simulink model "hw2Q6_model"  (R2021a)
settings: Solver=VariableStepAuto  StartTime=0.0  StopTime=time_end  RelTol=1e-3
settings Model: Creator=kaiyu  LastModifiedBy=kaiyu

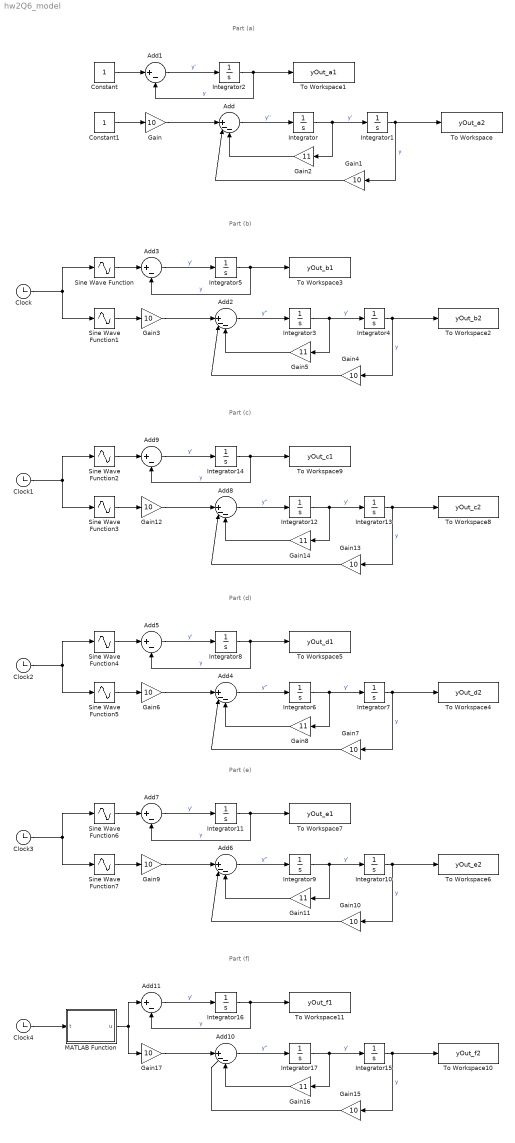
== system hw2Q6_model ==
  note: Part (a)
  note: Part (b)
  note: Part (d)
  note: Part (e)
  note: Part (c)
  note: Part (f)
  Add{,2,4,6,8,10} (6 alike) : Sum  Inputs=||+--
  Add{1,3,5,7,9,11} (6 alike) : Sum  Inputs=|+-
  Clock{,1..4} (5 alike) : Clock
  Constant : Constant
  Constant1 : Constant
  Gain{,1,3..4,6..7,9..10,12..13,15,17} (12 alike) : Gain  Gain=10
  Gain{2,5,8,11,14,16} (6 alike) : Gain  Gain=11
  Integrator{,1..17} (18 alike) : Integrator
  MATLAB Function : MATLAB Function  TreatAsAtomicUnit=on
  Sine Wave Function : Sin  TimeSource=Use external signal  SampleTime=0
  Sine Wave Function1 : Sin  TimeSource=Use external signal  SampleTime=0
  Sine Wave Function2 : Sin  TimeSource=Use external signal  Frequency=5  Phase=pi / 2  SampleTime=0
  Sine Wave Function3 : Sin  TimeSource=Use external signal  Frequency=5  Phase=pi / 2  SampleTime=0
  Sine Wave Function4 : Sin  TimeSource=Use external signal  Amplitude=25  Frequency=10  Phase=pi / 2  SampleTime=0
  Sine Wave Function5 : Sin  TimeSource=Use external signal  Amplitude=25  Frequency=10  Phase=pi / 2  SampleTime=0
  Sine Wave Function6 : Sin  TimeSource=Use external signal  Amplitude=25  Frequency=20  Phase=pi / 2  SampleTime=0
  Sine Wave Function7 : Sin  TimeSource=Use external signal  Amplitude=25  Frequency=20  Phase=pi / 2  SampleTime=0
  To Workspace : ToWorkspace  VariableName=yOut_a2  SaveFormat=Timeseries  SampleTime=-1
  To Workspace1 : ToWorkspace  VariableName=yOut_a1  SaveFormat=Timeseries  SampleTime=-1
  To Workspace10 : ToWorkspace  VariableName=yOut_f2  SaveFormat=Timeseries  SampleTime=-1
  To Workspace11 : ToWorkspace  VariableName=yOut_f1  SaveFormat=Timeseries  SampleTime=-1
  To Workspace2 : ToWorkspace  VariableName=yOut_b2  SaveFormat=Timeseries  SampleTime=-1
  To Workspace3 : ToWorkspace  VariableName=yOut_b1  SaveFormat=Timeseries  SampleTime=-1
  To Workspace4 : ToWorkspace  VariableName=yOut_d2  SaveFormat=Timeseries  SampleTime=-1
  To Workspace5 : ToWorkspace  VariableName=yOut_d1  SaveFormat=Timeseries  SampleTime=-1
  To Workspace6 : ToWorkspace  VariableName=yOut_e2  SaveFormat=Timeseries  SampleTime=-1
  To Workspace7 : ToWorkspace  VariableName=yOut_e1  SaveFormat=Timeseries  SampleTime=-1
  To Workspace8 : ToWorkspace  VariableName=yOut_c2  SaveFormat=Timeseries  SampleTime=-1
  To Workspace9 : ToWorkspace  VariableName=yOut_c1  SaveFormat=Timeseries  SampleTime=-1
  wires:
  Gain/1 -> Add/1
  Add/1 -> Integrator/1  "y''"
  Integrator/1 -> Gain2/1, Integrator1/1  "y'"
  Integrator1/1 -> Gain1/1, To Workspace/1  "y"
  Gain1/1 -> Add/2
  Gain2/1 -> Add/3
  Add1/1 -> Integrator2/1  "y'"
  Integrator2/1 -> Add1/2, To Workspace1/1  "y"
  Add3/1 -> Integrator5/1  "y'"
  Gain5/1 -> Add2/3
  Integrator4/1 -> Gain4/1, To Workspace2/1  "y"
  Integrator5/1 -> Add3/2, To Workspace3/1  "y"
  Gain4/1 -> Add2/2
  Gain3/1 -> Add2/1
  Integrator3/1 -> Gain5/1, Integrator4/1  "y'"
  Add2/1 -> Integrator3/1  "y''"
  Constant/1 -> Add1/1
  Constant1/1 -> Gain/1
  Gain7/1 -> Add4/2
  Integrator6/1 -> Gain8/1, Integrator7/1  "y'"
  Gain6/1 -> Add4/1
  Integrator8/1 -> Add5/2, To Workspace5/1  "y"
  Add4/1 -> Integrator6/1  "y''"
  Integrator7/1 -> Gain7/1, To Workspace4/1  "y"
  Gain8/1 -> Add4/3
  Add5/1 -> Integrator8/1  "y'"
  Add6/1 -> Integrator9/1  "y''"
  Integrator11/1 -> Add7/2, To Workspace7/1  "y"
  Gain9/1 -> Add6/1
  Add7/1 -> Integrator11/1  "y'"
  Gain10/1 -> Add6/2
  Integrator10/1 -> Gain10/1, To Workspace6/1  "y"
  Integrator9/1 -> Gain11/1, Integrator10/1  "y'"
  Gain11/1 -> Add6/3
  Add8/1 -> Integrator12/1  "y''"
  Integrator14/1 -> Add9/2, To Workspace9/1  "y"
  Gain12/1 -> Add8/1
  Add9/1 -> Integrator14/1  "y'"
  Gain13/1 -> Add8/2
  Integrator13/1 -> Gain13/1, To Workspace8/1  "y"
  Integrator12/1 -> Gain14/1, Integrator13/1  "y'"
  Gain14/1 -> Add8/3
  Integrator17/1 -> Gain16/1, Integrator15/1  "y'"
  Gain16/1 -> Add10/3
  Integrator15/1 -> Gain15/1, To Workspace10/1  "y"
  Gain17/1 -> Add10/1
  Add11/1 -> Integrator16/1  "y'"
  Integrator16/1 -> Add11/2, To Workspace11/1  "y"
  Gain15/1 -> Add10/2
  Add10/1 -> Integrator17/1  "y''"
  Sine Wave Function/1 -> Add3/1
  Sine Wave Function1/1 -> Gain3/1
  Clock/1 -> Sine Wave Function/1, Sine Wave Function1/1
  Sine Wave Function2/1 -> Add9/1
  Sine Wave Function3/1 -> Gain12/1
  Clock1/1 -> Sine Wave Function2/1, Sine Wave Function3/1
  Sine Wave Function4/1 -> Add5/1
  Sine Wave Function5/1 -> Gain6/1
  Clock2/1 -> Sine Wave Function5/1, Sine Wave Function4/1
  Sine Wave Function6/1 -> Add7/1
  Sine Wave Function7/1 -> Gain9/1
  Clock3/1 -> Sine Wave Function7/1, Sine Wave Function6/1
  MATLAB Function/1(u) -> Add11/1, Gain17/1
  Clock4/1 -> MATLAB Function/1(t)

== matlab function hw2Q6_model/MATLAB Function ==
  data: t input; u output
function u = hw2Q6_f_func(t)
if (0 <= t) && (t < 3)
    input = t;

elseif (3 <= t) && (t < 5)
    input = 3;

elseif (5 <= t) && (t < 7)
    input = -3;
    
else
    input = 2 * t - 17;
end

u = input;
